simulink model "D_20210914_Modell_Inbetriebnahme_BreakOutBox_Jetson"  (R2021a)
(part 5 of 7)

  CAN Unpack60/8 -> Terminator530/1
  CAN Unpack60/11 -> Bus Creator60/4  "RCS"
  CAN Unpack60/14 -> Terminator533/1
  CAN Unpack60/15 -> Bus Creator60/6  "Speed_Radial"
  CAN Unpack60/9 -> Terminator531/1
  CAN Unpack60/6 -> Terminator528/1
  CAN Unpack60/16 -> Bus Creator60/7  "CAN ID"
  CAN Unpack60/17 -> Bus Creator60/8  "Timestamp"
  Bus Creator60/1 -> Bus Creator1/60  "Data_059"
  CAN Unpack60/1 -> Bus Creator60/1  "AZ_Winkel"
  CAN Unpack61/3 -> Terminator534/1
  CAN Unpack61/2 -> Bus Creator61/2  "EL_Angle"
  CAN Unpack61/13 -> Terminator541/1
  CAN Unpack61/7 -> Terminator538/1
  CAN Unpack61/12 -> Bus Creator61/5  "Range"
  CAN Unpack61/10 -> Bus Creator61/3  "Mode_Signal"
  CAN Unpack61/4 -> Terminator535/1
  CAN Unpack61/5 -> Terminator536/1
  CAN Unpack61/8 -> Terminator539/1
  CAN Unpack61/11 -> Bus Creator61/4  "RCS"
  CAN Unpack61/14 -> Terminator542/1
  CAN Unpack61/15 -> Bus Creator61/6  "Speed_Radial"
  CAN Unpack61/9 -> Terminator540/1
  CAN Unpack61/6 -> Terminator537/1
  CAN Unpack61/16 -> Bus Creator61/7  "CAN ID"
  CAN Unpack61/17 -> Bus Creator61/8  "Timestamp"
  Bus Creator61/1 -> Bus Creator1/61  "Data_060"
  CAN Unpack61/1 -> Bus Creator61/1  "AZ_Winkel"
  CAN Unpack62/3 -> Terminator543/1
  CAN Unpack62/2 -> Bus Creator62/2  "EL_Angle"
  CAN Unpack62/13 -> Terminator550/1
  CAN Unpack62/7 -> Terminator547/1
  CAN Unpack62/12 -> Bus Creator62/5  "Range"
  CAN Unpack62/10 -> Bus Creator62/3  "Mode_Signal"
  CAN Unpack62/4 -> Terminator544/1
  CAN Unpack62/5 -> Terminator545/1
  CAN Unpack62/8 -> Terminator548/1
  CAN Unpack62/11 -> Bus Creator62/4  "RCS"
  CAN Unpack62/14 -> Terminator551/1
  CAN Unpack62/15 -> Bus Creator62/6  "Speed_Radial"
  CAN Unpack62/9 -> Terminator549/1
  CAN Unpack62/6 -> Terminator546/1
  CAN Unpack62/16 -> Bus Creator62/7  "CAN ID"
  CAN Unpack62/17 -> Bus Creator62/8  "Timestamp"
  Bus Creator62/1 -> Bus Creator1/62  "Data_061"
  CAN Unpack62/1 -> Bus Creator62/1  "AZ_Winkel"
  CAN Unpack63/3 -> Terminator552/1
  CAN Unpack63/2 -> Bus Creator63/2  "EL_Angle"
  CAN Unpack63/13 -> Terminator559/1
  CAN Unpack63/7 -> Terminator556/1
  CAN Unpack63/12 -> Bus Creator63/5  "Range"
  CAN Unpack63/10 -> Bus Creator63/3  "Mode_Signal"
  CAN Unpack63/4 -> Terminator553/1
  CAN Unpack63/5 -> Terminator554/1
  CAN Unpack63/8 -> Terminator557/1
  CAN Unpack63/11 -> Bus Creator63/4  "RCS"
  CAN Unpack63/14 -> Terminator560/1
  CAN Unpack63/15 -> Bus Creator63/6  "Speed_Radial"
  CAN Unpack63/9 -> Terminator558/1
  CAN Unpack63/6 -> Terminator555/1
  CAN Unpack63/16 -> Bus Creator63/7  "CAN ID"
  CAN Unpack63/17 -> Bus Creator63/8  "Timestamp"
  Bus Creator63/1 -> Bus Creator1/63  "Data_062"
  CAN Unpack63/1 -> Bus Creator63/1  "AZ_Winkel"
  CAN Unpack64/3 -> Terminator561/1
  CAN Unpack64/2 -> Bus Creator64/2  "EL_Angle"
  CAN Unpack64/13 -> Terminator568/1
  CAN Unpack64/7 -> Terminator565/1
  CAN Unpack64/12 -> Bus Creator64/5  "Range"
  CAN Unpack64/10 -> Bus Creator64/3  "Mode_Signal"
  CAN Unpack64/4 -> Terminator562/1
  CAN Unpack64/5 -> Terminator563/1
  CAN Unpack64/8 -> Terminator566/1
  CAN Unpack64/11 -> Bus Creator64/4  "RCS"
  CAN Unpack64/14 -> Terminator569/1
  CAN Unpack64/15 -> Bus Creator64/6  "Speed_Radial"
  CAN Unpack64/9 -> Terminator567/1
  CAN Unpack64/6 -> Terminator564/1
  CAN Unpack64/16 -> Bus Creator64/7  "CAN ID"
  CAN Unpack64/17 -> Bus Creator64/8  "Timestamp"
  Bus Creator64/1 -> Bus Creator1/64  "Data_063"
  CAN Unpack64/1 -> Bus Creator64/1  "AZ_Winkel"
  CAN Unpack65/3 -> Terminator570/1
  CAN Unpack65/2 -> Bus Creator65/2  "EL_Angle"
  CAN Unpack65/13 -> Terminator577/1
  CAN Unpack65/7 -> Terminator574/1
  CAN Unpack65/12 -> Bus Creator65/5  "Range"
  CAN Unpack65/10 -> Bus Creator65/3  "Mode_Signal"
  CAN Unpack65/4 -> Terminator571/1
  CAN Unpack65/5 -> Terminator572/1
  CAN Unpack65/8 -> Terminator575/1
  CAN Unpack65/11 -> Bus Creator65/4  "RCS"
  CAN Unpack65/14 -> Terminator578/1
  CAN Unpack65/15 -> Bus Creator65/6  "Speed_Radial"
  CAN Unpack65/9 -> Terminator576/1
  CAN Unpack65/6 -> Terminator573/1
  CAN Unpack65/16 -> Bus Creator65/7  "CAN ID"
  CAN Unpack65/17 -> Bus Creator65/8  "Timestamp"
  Bus Creator65/1 -> Bus Creator1/65  "Data_064"
  CAN Unpack65/1 -> Bus Creator65/1  "AZ_Winkel"
  CAN Unpack66/3 -> Terminator579/1
  CAN Unpack66/2 -> Bus Creator66/2  "EL_Angle"
  CAN Unpack66/13 -> Terminator586/1
  CAN Unpack66/7 -> Terminator583/1
  CAN Unpack66/12 -> Bus Creator66/5  "Range"
  CAN Unpack66/10 -> Bus Creator66/3  "Mode_Signal"
  CAN Unpack66/4 -> Terminator580/1
  CAN Unpack66/5 -> Terminator581/1
  CAN Unpack66/8 -> Terminator584/1
  CAN Unpack66/11 -> Bus Creator66/4  "RCS"
  CAN Unpack66/14 -> Terminator587/1
  CAN Unpack66/15 -> Bus Creator66/6  "Speed_Radial"
  CAN Unpack66/9 -> Terminator585/1
  CAN Unpack66/6 -> Terminator582/1
  CAN Unpack66/16 -> Bus Creator66/7  "CAN ID"
  CAN Unpack66/17 -> Bus Creator66/8  "Timestamp"
  Bus Creator66/1 -> Bus Creator1/66  "Data_065"
  CAN Unpack66/1 -> Bus Creator66/1  "AZ_Winkel"
  CAN Unpack67/3 -> Terminator588/1
  CAN Unpack67/2 -> Bus Creator67/2  "EL_Angle"
  CAN Unpack67/13 -> Terminator595/1
  CAN Unpack67/7 -> Terminator592/1
  CAN Unpack67/12 -> Bus Creator67/5  "Range"
  CAN Unpack67/10 -> Bus Creator67/3  "Mode_Signal"
  CAN Unpack67/4 -> Terminator589/1
  CAN Unpack67/5 -> Terminator590/1
  CAN Unpack67/8 -> Terminator593/1
  CAN Unpack67/11 -> Bus Creator67/4  "RCS"
  CAN Unpack67/14 -> Terminator596/1
  CAN Unpack67/15 -> Bus Creator67/6  "Speed_Radial"
  CAN Unpack67/9 -> Terminator594/1
  CAN Unpack67/6 -> Terminator591/1
  CAN Unpack67/16 -> Bus Creator67/7  "CAN ID"
  CAN Unpack67/17 -> Bus Creator67/8  "Timestamp"
  Bus Creator67/1 -> Bus Creator1/67  "Data_066"
  CAN Unpack67/1 -> Bus Creator67/1  "AZ_Winkel"
  CAN Unpack68/3 -> Terminator597/1
  CAN Unpack68/2 -> Bus Creator68/2  "EL_Angle"
  CAN Unpack68/13 -> Terminator604/1
  CAN Unpack68/7 -> Terminator601/1
  CAN Unpack68/12 -> Bus Creator68/5  "Range"
  CAN Unpack68/10 -> Bus Creator68/3  "Mode_Signal"
  CAN Unpack68/4 -> Terminator598/1
  CAN Unpack68/5 -> Terminator599/1
  CAN Unpack68/8 -> Terminator602/1
  CAN Unpack68/11 -> Bus Creator68/4  "RCS"
  CAN Unpack68/14 -> Terminator605/1
  CAN Unpack68/15 -> Bus Creator68/6  "Speed_Radial"
  CAN Unpack68/9 -> Terminator603/1
  CAN Unpack68/6 -> Terminator600/1
  CAN Unpack68/16 -> Bus Creator68/7  "CAN ID"
  CAN Unpack68/17 -> Bus Creator68/8  "Timestamp"
  Bus Creator68/1 -> Bus Creator1/68  "Data_067"
  CAN Unpack68/1 -> Bus Creator68/1  "AZ_Winkel"
  CAN Unpack69/3 -> Terminator606/1
  CAN Unpack69/2 -> Bus Creator69/2  "EL_Angle"
  CAN Unpack69/13 -> Terminator613/1
  CAN Unpack69/7 -> Terminator610/1
  CAN Unpack69/12 -> Bus Creator69/5  "Range"
  CAN Unpack69/10 -> Bus Creator69/3  "Mode_Signal"
  CAN Unpack69/4 -> Terminator607/1
  CAN Unpack69/5 -> Terminator608/1
  CAN Unpack69/8 -> Terminator611/1
  CAN Unpack69/11 -> Bus Creator69/4  "RCS"
  CAN Unpack69/14 -> Terminator614/1
  CAN Unpack69/15 -> Bus Creator69/6  "Speed_Radial"
  CAN Unpack69/9 -> Terminator612/1
  CAN Unpack69/6 -> Terminator609/1
  CAN Unpack69/16 -> Bus Creator69/7  "CAN ID"
  CAN Unpack69/17 -> Bus Creator69/8  "Timestamp"
  Bus Creator69/1 -> Bus Creator1/69  "Data_068"
  CAN Unpack69/1 -> Bus Creator69/1  "AZ_Winkel"
  CAN Unpack70/3 -> Terminator615/1
  CAN Unpack70/2 -> Bus Creator70/2  "EL_Angle"
  CAN Unpack70/13 -> Terminator622/1
  CAN Unpack70/7 -> Terminator619/1
  CAN Unpack70/12 -> Bus Creator70/5  "Range"
  CAN Unpack70/10 -> Bus Creator70/3  "Mode_Signal"
  CAN Unpack70/4 -> Terminator616/1
  CAN Unpack70/5 -> Terminator617/1
  CAN Unpack70/8 -> Terminator620/1
  CAN Unpack70/11 -> Bus Creator70/4  "RCS"
  CAN Unpack70/14 -> Terminator623/1
  CAN Unpack70/15 -> Bus Creator70/6  "Speed_Radial"
  CAN Unpack70/9 -> Terminator621/1
  CAN Unpack70/6 -> Terminator618/1
  CAN Unpack70/16 -> Bus Creator70/7  "CAN ID"
  CAN Unpack70/17 -> Bus Creator70/8  "Timestamp"
  Bus Creator70/1 -> Bus Creator1/70  "Data_069"
  CAN Unpack70/1 -> Bus Creator70/1  "AZ_Winkel"
  CAN Unpack71/3 -> Terminator624/1
  CAN Unpack71/2 -> Bus Creator71/2  "EL_Angle"
  CAN Unpack71/13 -> Terminator631/1
  CAN Unpack71/7 -> Terminator628/1
  CAN Unpack71/12 -> Bus Creator71/5  "Range"
  CAN Unpack71/10 -> Bus Creator71/3  "Mode_Signal"
  CAN Unpack71/4 -> Terminator625/1
  CAN Unpack71/5 -> Terminator626/1
  CAN Unpack71/8 -> Terminator629/1
  CAN Unpack71/11 -> Bus Creator71/4  "RCS"
  CAN Unpack71/14 -> Terminator632/1
  CAN Unpack71/15 -> Bus Creator71/6  "Speed_Radial"
  CAN Unpack71/9 -> Terminator630/1
  CAN Unpack71/6 -> Terminator627/1
  CAN Unpack71/16 -> Bus Creator71/7  "CAN ID"
  CAN Unpack71/17 -> Bus Creator71/8  "Timestamp"
  Bus Creator71/1 -> Bus Creator1/71  "Data_070"
  CAN Unpack71/1 -> Bus Creator71/1  "AZ_Winkel"
  CAN Unpack72/3 -> Terminator633/1
  CAN Unpack72/2 -> Bus Creator72/2  "EL_Angle"
  CAN Unpack72/13 -> Terminator640/1
  CAN Unpack72/7 -> Terminator637/1
  CAN Unpack72/12 -> Bus Creator72/5  "Range"
  CAN Unpack72/10 -> Bus Creator72/3  "Mode_Signal"
  CAN Unpack72/4 -> Terminator634/1
  CAN Unpack72/5 -> Terminator635/1
  CAN Unpack72/8 -> Terminator638/1
  CAN Unpack72/11 -> Bus Creator72/4  "RCS"
  CAN Unpack72/14 -> Terminator641/1
  CAN Unpack72/15 -> Bus Creator72/6  "Speed_Radial"
  CAN Unpack72/9 -> Terminator639/1
  CAN Unpack72/6 -> Terminator636/1
  CAN Unpack72/16 -> Bus Creator72/7  "CAN ID"
  CAN Unpack72/17 -> Bus Creator72/8  "Timestamp"
  Bus Creator72/1 -> Bus Creator1/72  "Data_071"
  CAN Unpack72/1 -> Bus Creator72/1  "AZ_Winkel"
  CAN Unpack73/3 -> Terminator642/1
  CAN Unpack73/2 -> Bus Creator73/2  "EL_Angle"
  CAN Unpack73/13 -> Terminator649/1
  CAN Unpack73/7 -> Terminator646/1
  CAN Unpack73/12 -> Bus Creator73/5  "Range"
  CAN Unpack73/10 -> Bus Creator73/3  "Mode_Signal"
  CAN Unpack73/4 -> Terminator643/1
  CAN Unpack73/5 -> Terminator644/1
  CAN Unpack73/8 -> Terminator647/1
  CAN Unpack73/11 -> Bus Creator73/4  "RCS"
  CAN Unpack73/14 -> Terminator650/1
  CAN Unpack73/15 -> Bus Creator73/6  "Speed_Radial"
  CAN Unpack73/9 -> Terminator648/1
  CAN Unpack73/6 -> Terminator645/1
  CAN Unpack73/16 -> Bus Creator73/7  "CAN ID"
  CAN Unpack73/17 -> Bus Creator73/8  "Timestamp"
  Bus Creator73/1 -> Bus Creator1/73  "Data_072"
  CAN Unpack73/1 -> Bus Creator73/1  "AZ_Winkel"
  CAN Unpack74/3 -> Terminator651/1
  CAN Unpack74/2 -> Bus Creator74/2  "EL_Angle"
  CAN Unpack74/13 -> Terminator658/1
  CAN Unpack74/7 -> Terminator655/1
  CAN Unpack74/12 -> Bus Creator74/5  "Range"
  CAN Unpack74/10 -> Bus Creator74/3  "Mode_Signal"
  CAN Unpack74/4 -> Terminator652/1
  CAN Unpack74/5 -> Terminator653/1
  CAN Unpack74/8 -> Terminator656/1
  CAN Unpack74/11 -> Bus Creator74/4  "RCS"
  CAN Unpack74/14 -> Terminator659/1
  CAN Unpack74/15 -> Bus Creator74/6  "Speed_Radial"
  CAN Unpack74/9 -> Terminator657/1
  CAN Unpack74/6 -> Terminator654/1
  CAN Unpack74/16 -> Bus Creator74/7  "CAN ID"
  CAN Unpack74/17 -> Bus Creator74/8  "Timestamp"
  Bus Creator74/1 -> Bus Creator1/74  "Data_073"
  CAN Unpack74/1 -> Bus Creator74/1  "AZ_Winkel"
  CAN Unpack75/3 -> Terminator660/1
  CAN Unpack75/2 -> Bus Creator75/2  "EL_Angle"
  CAN Unpack75/13 -> Terminator667/1
  CAN Unpack75/7 -> Terminator664/1
  CAN Unpack75/12 -> Bus Creator75/5  "Range"
  CAN Unpack75/10 -> Bus Creator75/3  "Mode_Signal"
  CAN Unpack75/4 -> Terminator661/1
  CAN Unpack75/5 -> Terminator662/1
  CAN Unpack75/8 -> Terminator665/1
  CAN Unpack75/11 -> Bus Creator75/4  "RCS"
  CAN Unpack75/14 -> Terminator668/1
  CAN Unpack75/15 -> Bus Creator75/6  "Speed_Radial"
  CAN Unpack75/9 -> Terminator666/1
  CAN Unpack75/6 -> Terminator663/1
  CAN Unpack75/16 -> Bus Creator75/7  "CAN ID"
  CAN Unpack75/17 -> Bus Creator75/8  "Timestamp"
  Bus Creator75/1 -> Bus Creator1/75  "Data_074"
  CAN Unpack75/1 -> Bus Creator75/1  "AZ_Winkel"
  CAN Unpack76/3 -> Terminator669/1
  CAN Unpack76/2 -> Bus Creator76/2  "EL_Angle"
  CAN Unpack76/13 -> Terminator676/1
  CAN Unpack76/7 -> Terminator673/1
  CAN Unpack76/12 -> Bus Creator76/5  "Range"
  CAN Unpack76/10 -> Bus Creator76/3  "Mode_Signal"
  CAN Unpack76/4 -> Terminator670/1
  CAN Unpack76/5 -> Terminator671/1
  CAN Unpack76/8 -> Terminator674/1
  CAN Unpack76/11 -> Bus Creator76/4  "RCS"
  CAN Unpack76/14 -> Terminator677/1
  CAN Unpack76/15 -> Bus Creator76/6  "Speed_Radial"
  CAN Unpack76/9 -> Terminator675/1
  CAN Unpack76/6 -> Terminator672/1
  CAN Unpack76/16 -> Bus Creator76/7  "CAN ID"
  CAN Unpack76/17 -> Bus Creator76/8  "Timestamp"
  Bus Creator76/1 -> Bus Creator1/76  "Data_075"
  CAN Unpack76/1 -> Bus Creator76/1  "AZ_Winkel"
  CAN Unpack77/3 -> Terminator678/1
  CAN Unpack77/2 -> Bus Creator77/2  "EL_Angle"
  CAN Unpack77/13 -> Terminator685/1
  CAN Unpack77/7 -> Terminator682/1
  CAN Unpack77/12 -> Bus Creator77/5  "Range"
  CAN Unpack77/10 -> Bus Creator77/3  "Mode_Signal"
  CAN Unpack77/4 -> Terminator679/1
  CAN Unpack77/5 -> Terminator680/1
  CAN Unpack77/8 -> Terminator683/1
  CAN Unpack77/11 -> Bus Creator77/4  "RCS"
  CAN Unpack77/14 -> Terminator686/1
  CAN Unpack77/15 -> Bus Creator77/6  "Speed_Radial"
  CAN Unpack77/9 -> Terminator684/1
  CAN Unpack77/6 -> Terminator681/1
  CAN Unpack77/16 -> Bus Creator77/7  "CAN ID"
  CAN Unpack77/17 -> Bus Creator77/8  "Timestamp"
  Bus Creator77/1 -> Bus Creator1/77  "Data_076"
  CAN Unpack77/1 -> Bus Creator77/1  "AZ_Winkel"
  CAN Unpack78/3 -> Terminator687/1
  CAN Unpack78/2 -> Bus Creator78/2  "EL_Angle"
  CAN Unpack78/13 -> Terminator694/1
  CAN Unpack78/7 -> Terminator691/1
  CAN Unpack78/12 -> Bus Creator78/5  "Range"
  CAN Unpack78/10 -> Bus Creator78/3  "Mode_Signal"
  CAN Unpack78/4 -> Terminator688/1
  CAN Unpack78/5 -> Terminator689/1
  CAN Unpack78/8 -> Terminator692/1
  CAN Unpack78/11 -> Bus Creator78/4  "RCS"
  CAN Unpack78/14 -> Terminator695/1
  CAN Unpack78/15 -> Bus Creator78/6  "Speed_Radial"
  CAN Unpack78/9 -> Terminator693/1
  CAN Unpack78/6 -> Terminator690/1
  CAN Unpack78/16 -> Bus Creator78/7  "CAN ID"
  CAN Unpack78/17 -> Bus Creator78/8  "Timestamp"
  Bus Creator78/1 -> Bus Creator1/78  "Data_077"
  CAN Unpack78/1 -> Bus Creator78/1  "AZ_Winkel"
  CAN Unpack79/3 -> Terminator696/1
  CAN Unpack79/2 -> Bus Creator79/2  "EL_Angle"
  CAN Unpack79/13 -> Terminator703/1
  CAN Unpack79/7 -> Terminator700/1
  CAN Unpack79/12 -> Bus Creator79/5  "Range"
  CAN Unpack79/10 -> Bus Creator79/3  "Mode_Signal"
  CAN Unpack79/4 -> Terminator697/1
  CAN Unpack79/5 -> Terminator698/1
  CAN Unpack79/8 -> Terminator701/1
  CAN Unpack79/11 -> Bus Creator79/4  "RCS"
  CAN Unpack79/14 -> Terminator704/1
  CAN Unpack79/15 -> Bus Creator79/6  "Speed_Radial"
  CAN Unpack79/9 -> Terminator702/1
  CAN Unpack79/6 -> Terminator699/1
  CAN Unpack79/16 -> Bus Creator79/7  "CAN ID"
  CAN Unpack79/17 -> Bus Creator79/8  "Timestamp"
  Bus Creator79/1 -> Bus Creator1/79  "Data_078"
  CAN Unpack79/1 -> Bus Creator79/1  "AZ_Winkel"
  CAN Unpack80/3 -> Terminator705/1
  CAN Unpack80/2 -> Bus Creator80/2  "EL_Angle"
  CAN Unpack80/13 -> Terminator712/1
  CAN Unpack80/7 -> Terminator709/1
  CAN Unpack80/12 -> Bus Creator80/5  "Range"
  CAN Unpack80/10 -> Bus Creator80/3  "Mode_Signal"
  CAN Unpack80/4 -> Terminator706/1
  CAN Unpack80/5 -> Terminator707/1
  CAN Unpack80/8 -> Terminator710/1
  CAN Unpack80/11 -> Bus Creator80/4  "RCS"
  CAN Unpack80/14 -> Terminator713/1
  CAN Unpack80/15 -> Bus Creator80/6  "Speed_Radial"
  CAN Unpack80/9 -> Terminator711/1
  CAN Unpack80/6 -> Terminator708/1
  CAN Unpack80/16 -> Bus Creator80/7  "CAN ID"
  CAN Unpack80/17 -> Bus Creator80/8  "Timestamp"
  Bus Creator80/1 -> Bus Creator1/80  "Data_079"
  CAN Unpack80/1 -> Bus Creator80/1  "AZ_Winkel"
  CAN Unpack81/3 -> Terminator714/1
  CAN Unpack81/2 -> Bus Creator81/2  "EL_Angle"
  CAN Unpack81/13 -> Terminator721/1
  CAN Unpack81/7 -> Terminator718/1
  CAN Unpack81/12 -> Bus Creator81/5  "Range"
  CAN Unpack81/10 -> Bus Creator81/3  "Mode_Signal"
  CAN Unpack81/4 -> Terminator715/1
  CAN Unpack81/5 -> Terminator716/1
  CAN Unpack81/8 -> Terminator719/1
  CAN Unpack81/11 -> Bus Creator81/4  "RCS"
  CAN Unpack81/14 -> Terminator722/1
  CAN Unpack81/15 -> Bus Creator81/6  "Speed_Radial"
  CAN Unpack81/9 -> Terminator720/1
  CAN Unpack81/6 -> Terminator717/1
  CAN Unpack81/16 -> Bus Creator81/7  "CAN ID"
  CAN Unpack81/17 -> Bus Creator81/8  "Timestamp"
  Bus Creator81/1 -> Bus Creator1/81  "Data_080"
  CAN Unpack81/1 -> Bus Creator81/1  "AZ_Winkel"
  CAN Unpack82/3 -> Terminator723/1
  CAN Unpack82/2 -> Bus Creator82/2  "EL_Angle"
  CAN Unpack82/13 -> Terminator730/1
  CAN Unpack82/7 -> Terminator727/1
  CAN Unpack82/12 -> Bus Creator82/5  "Range"
  CAN Unpack82/10 -> Bus Creator82/3  "Mode_Signal"
  CAN Unpack82/4 -> Terminator724/1
  CAN Unpack82/5 -> Terminator725/1
  CAN Unpack82/8 -> Terminator728/1
  CAN Unpack82/11 -> Bus Creator82/4  "RCS"
  CAN Unpack82/14 -> Terminator731/1
  CAN Unpack82/15 -> Bus Creator82/6  "Speed_Radial"
  CAN Unpack82/9 -> Terminator729/1
  CAN Unpack82/6 -> Terminator726/1
  CAN Unpack82/16 -> Bus Creator82/7  "CAN ID"
  CAN Unpack82/17 -> Bus Creator82/8  "Timestamp"
  Bus Creator82/1 -> Bus Creator1/82  "Data_081"
  CAN Unpack82/1 -> Bus Creator82/1  "AZ_Winkel"
  CAN Unpack83/3 -> Terminator732/1
  CAN Unpack83/2 -> Bus Creator83/2  "EL_Angle"
  CAN Unpack83/13 -> Terminator739/1
  CAN Unpack83/7 -> Terminator736/1
  CAN Unpack83/12 -> Bus Creator83/5  "Range"
  CAN Unpack83/10 -> Bus Creator83/3  "Mode_Signal"
  CAN Unpack83/4 -> Terminator733/1
  CAN Unpack83/5 -> Terminator734/1
  CAN Unpack83/8 -> Terminator737/1
  CAN Unpack83/11 -> Bus Creator83/4  "RCS"
  CAN Unpack83/14 -> Terminator740/1
  CAN Unpack83/15 -> Bus Creator83/6  "Speed_Radial"
  CAN Unpack83/9 -> Terminator738/1
  CAN Unpack83/6 -> Terminator735/1
  CAN Unpack83/16 -> Bus Creator83/7  "CAN ID"
  CAN Unpack83/17 -> Bus Creator83/8  "Timestamp"
  Bus Creator83/1 -> Bus Creator1/83  "Data_082"
  CAN Unpack83/1 -> Bus Creator83/1  "AZ_Winkel"
  CAN Unpack84/3 -> Terminator741/1
  CAN Unpack84/2 -> Bus Creator84/2  "EL_Angle"
  CAN Unpack84/13 -> Terminator748/1
  CAN Unpack84/7 -> Terminator745/1
  CAN Unpack84/12 -> Bus Creator84/5  "Range"
  CAN Unpack84/10 -> Bus Creator84/3  "Mode_Signal"
  CAN Unpack84/4 -> Terminator742/1
  CAN Unpack84/5 -> Terminator743/1
  CAN Unpack84/8 -> Terminator746/1
  CAN Unpack84/11 -> Bus Creator84/4  "RCS"
  CAN Unpack84/14 -> Terminator749/1
  CAN Unpack84/15 -> Bus Creator84/6  "Speed_Radial"
  CAN Unpack84/9 -> Terminator747/1
  CAN Unpack84/6 -> Terminator744/1
  CAN Unpack84/16 -> Bus Creator84/7  "CAN ID"
  CAN Unpack84/17 -> Bus Creator84/8  "Timestamp"
  Bus Creator84/1 -> Bus Creator1/84  "Data_083"
  CAN Unpack84/1 -> Bus Creator84/1  "AZ_Winkel"
  CAN Unpack85/3 -> Terminator750/1
  CAN Unpack85/2 -> Bus Creator85/2  "EL_Angle"
  CAN Unpack85/13 -> Terminator757/1
  CAN Unpack85/7 -> Terminator754/1
  CAN Unpack85/12 -> Bus Creator85/5  "Range"
  CAN Unpack85/10 -> Bus Creator85/3  "Mode_Signal"
  CAN Unpack85/4 -> Terminator751/1
  CAN Unpack85/5 -> Terminator752/1
  CAN Unpack85/8 -> Terminator755/1
  CAN Unpack85/11 -> Bus Creator85/4  "RCS"
  CAN Unpack85/14 -> Terminator758/1
  CAN Unpack85/15 -> Bus Creator85/6  "Speed_Radial"
  CAN Unpack85/9 -> Terminator756/1
  CAN Unpack85/6 -> Terminator753/1
  CAN Unpack85/16 -> Bus Creator85/7  "CAN ID"
  CAN Unpack85/17 -> Bus Creator85/8  "Timestamp"
  Bus Creator85/1 -> Bus Creator1/85  "Data_084"
  CAN Unpack85/1 -> Bus Creator85/1  "AZ_Winkel"
  CAN Unpack86/3 -> Terminator759/1
  CAN Unpack86/2 -> Bus Creator86/2  "EL_Angle"
  CAN Unpack86/13 -> Terminator766/1
  CAN Unpack86/7 -> Terminator763/1
  CAN Unpack86/12 -> Bus Creator86/5  "Range"
  CAN Unpack86/10 -> Bus Creator86/3  "Mode_Signal"
  CAN Unpack86/4 -> Terminator760/1
  CAN Unpack86/5 -> Terminator761/1
  CAN Unpack86/8 -> Terminator764/1
  CAN Unpack86/11 -> Bus Creator86/4  "RCS"
  CAN Unpack86/14 -> Terminator767/1
  CAN Unpack86/15 -> Bus Creator86/6  "Speed_Radial"
  CAN Unpack86/9 -> Terminator765/1
  CAN Unpack86/6 -> Terminator762/1
  CAN Unpack86/16 -> Bus Creator86/7  "CAN ID"
  CAN Unpack86/17 -> Bus Creator86/8  "Timestamp"
  Bus Creator86/1 -> Bus Creator1/86  "Data_085"
  CAN Unpack86/1 -> Bus Creator86/1  "AZ_Winkel"
  CAN Unpack87/3 -> Terminator768/1
  CAN Unpack87/2 -> Bus Creator87/2  "EL_Angle"
  CAN Unpack87/13 -> Terminator775/1
  CAN Unpack87/7 -> Terminator772/1
  CAN Unpack87/12 -> Bus Creator87/5  "Range"
  CAN Unpack87/10 -> Bus Creator87/3  "Mode_Signal"
  CAN Unpack87/4 -> Terminator769/1
  CAN Unpack87/5 -> Terminator770/1
  CAN Unpack87/8 -> Terminator773/1
  CAN Unpack87/11 -> Bus Creator87/4  "RCS"
  CAN Unpack87/14 -> Terminator776/1
  CAN Unpack87/15 -> Bus Creator87/6  "Speed_Radial"
  CAN Unpack87/9 -> Terminator774/1
  CAN Unpack87/6 -> Terminator771/1
  CAN Unpack87/16 -> Bus Creator87/7  "CAN ID"
  CAN Unpack87/17 -> Bus Creator87/8  "Timestamp"
  Bus Creator87/1 -> Bus Creator1/87  "Data_086"
  CAN Unpack87/1 -> Bus Creator87/1  "AZ_Winkel"
  CAN Unpack88/3 -> Terminator777/1
  CAN Unpack88/2 -> Bus Creator88/2  "EL_Angle"
  CAN Unpack88/13 -> Terminator784/1
  CAN Unpack88/7 -> Terminator781/1
  CAN Unpack88/12 -> Bus Creator88/5  "Range"
  CAN Unpack88/10 -> Bus Creator88/3  "Mode_Signal"
  CAN Unpack88/4 -> Terminator778/1
  CAN Unpack88/5 -> Terminator779/1
  CAN Unpack88/8 -> Terminator782/1
  CAN Unpack88/11 -> Bus Creator88/4  "RCS"
  CAN Unpack88/14 -> Terminator785/1
  CAN Unpack88/15 -> Bus Creator88/6  "Speed_Radial"
  CAN Unpack88/9 -> Terminator783/1
  CAN Unpack88/6 -> Terminator780/1
  CAN Unpack88/16 -> Bus Creator88/7  "CAN ID"
  CAN Unpack88/17 -> Bus Creator88/8  "Timestamp"
  Bus Creator88/1 -> Bus Creator1/88  "Data_087"
  CAN Unpack88/1 -> Bus Creator88/1  "AZ_Winkel"
  CAN Unpack89/3 -> Terminator786/1
  CAN Unpack89/2 -> Bus Creator89/2  "EL_Angle"
  CAN Unpack89/13 -> Terminator793/1
  CAN Unpack89/7 -> Terminator790/1
  CAN Unpack89/12 -> Bus Creator89/5  "Range"
  CAN Unpack89/10 -> Bus Creator89/3  "Mode_Signal"
  CAN Unpack89/4 -> Terminator787/1
  CAN Unpack89/5 -> Terminator788/1
  CAN Unpack89/8 -> Terminator791/1
  CAN Unpack89/11 -> Bus Creator89/4  "RCS"
  CAN Unpack89/14 -> Terminator794/1
  CAN Unpack89/15 -> Bus Creator89/6  "Speed_Radial"
  CAN Unpack89/9 -> Terminator792/1
  CAN Unpack89/6 -> Terminator789/1
  CAN Unpack89/16 -> Bus Creator89/7  "CAN ID"
  CAN Unpack89/17 -> Bus Creator89/8  "Timestamp"
  Bus Creator89/1 -> Bus Creator1/89  "Data_088"
  CAN Unpack89/1 -> Bus Creator89/1  "AZ_Winkel"
  CAN Unpack90/3 -> Terminator795/1
  CAN Unpack90/2 -> Bus Creator90/2  "EL_Angle"
  CAN Unpack90/13 -> Terminator802/1
  CAN Unpack90/7 -> Terminator799/1
  CAN Unpack90/12 -> Bus Creator90/5  "Range"
  CAN Unpack90/10 -> Bus Creator90/3  "Mode_Signal"
  CAN Unpack90/4 -> Terminator796/1
  CAN Unpack90/5 -> Terminator797/1
  CAN Unpack90/8 -> Terminator800/1
  CAN Unpack90/11 -> Bus Creator90/4  "RCS"
  CAN Unpack90/14 -> Terminator803/1
  CAN Unpack90/15 -> Bus Creator90/6  "Speed_Radial"
  CAN Unpack90/9 -> Terminator801/1
  CAN Unpack90/6 -> Terminator798/1
  CAN Unpack90/16 -> Bus Creator90/7  "CAN ID"
  CAN Unpack90/17 -> Bus Creator90/8  "Timestamp"
  Bus Creator90/1 -> Bus Creator1/90  "Data_089"
  CAN Unpack90/1 -> Bus Creator90/1  "AZ_Winkel"
  CAN Unpack91/3 -> Terminator804/1
  CAN Unpack91/2 -> Bus Creator91/2  "EL_Angle"
  CAN Unpack91/13 -> Terminator811/1
  CAN Unpack91/7 -> Terminator808/1
  CAN Unpack91/12 -> Bus Creator91/5  "Range"
  CAN Unpack91/10 -> Bus Creator91/3  "Mode_Signal"
  CAN Unpack91/4 -> Terminator805/1
  CAN Unpack91/5 -> Terminator806/1
  CAN Unpack91/8 -> Terminator809/1
  CAN Unpack91/11 -> Bus Creator91/4  "RCS"
  CAN Unpack91/14 -> Terminator812/1
  CAN Unpack91/15 -> Bus Creator91/6  "Speed_Radial"
  CAN Unpack91/9 -> Terminator810/1
  CAN Unpack91/6 -> Terminator807/1
  CAN Unpack91/16 -> Bus Creator91/7  "CAN ID"
  CAN Unpack91/17 -> Bus Creator91/8  "Timestamp"
  Bus Creator91/1 -> Bus Creator1/91  "Data_090"
  CAN Unpack91/1 -> Bus Creator91/1  "AZ_Winkel"
  CAN Unpack92/3 -> Terminator813/1
  CAN Unpack92/2 -> Bus Creator92/2  "EL_Angle"
  CAN Unpack92/13 -> Terminator820/1
  CAN Unpack92/7 -> Terminator817/1
  CAN Unpack92/12 -> Bus Creator92/5  "Range"
  CAN Unpack92/10 -> Bus Creator92/3  "Mode_Signal"
  CAN Unpack92/4 -> Terminator814/1
  CAN Unpack92/5 -> Terminator815/1
  CAN Unpack92/8 -> Terminator818/1
  CAN Unpack92/11 -> Bus Creator92/4  "RCS"
  CAN Unpack92/14 -> Terminator821/1
  CAN Unpack92/15 -> Bus Creator92/6  "Speed_Radial"
  CAN Unpack92/9 -> Terminator819/1
  CAN Unpack92/6 -> Terminator816/1
  CAN Unpack92/16 -> Bus Creator92/7  "CAN ID"
  CAN Unpack92/17 -> Bus Creator92/8  "Timestamp"
  Bus Creator92/1 -> Bus Creator1/92  "Data_091"
  CAN Unpack92/1 -> Bus Creator92/1  "AZ_Winkel"
  CAN Unpack93/3 -> Terminator822/1
  CAN Unpack93/2 -> Bus Creator93/2  "EL_Angle"
  CAN Unpack93/13 -> Terminator829/1
  CAN Unpack93/7 -> Terminator826/1
  CAN Unpack93/12 -> Bus Creator93/5  "Range"
  CAN Unpack93/10 -> Bus Creator93/3  "Mode_Signal"
  CAN Unpack93/4 -> Terminator823/1
  CAN Unpack93/5 -> Terminator824/1
  CAN Unpack93/8 -> Terminator827/1
  CAN Unpack93/11 -> Bus Creator93/4  "RCS"
  CAN Unpack93/14 -> Terminator830/1
  CAN Unpack93/15 -> Bus Creator93/6  "Speed_Radial"
  CAN Unpack93/9 -> Terminator828/1
  CAN Unpack93/6 -> Terminator825/1
  CAN Unpack93/16 -> Bus Creator93/7  "CAN ID"
  CAN Unpack93/17 -> Bus Creator93/8  "Timestamp"
  Bus Creator93/1 -> Bus Creator1/93  "Data_092"
  CAN Unpack93/1 -> Bus Creator93/1  "AZ_Winkel"
  CAN Unpack94/3 -> Terminator831/1
  CAN Unpack94/2 -> Bus Creator94/2  "EL_Angle"
  CAN Unpack94/13 -> Terminator838/1
  CAN Unpack94/7 -> Terminator835/1
  CAN Unpack94/12 -> Bus Creator94/5  "Range"
  CAN Unpack94/10 -> Bus Creator94/3  "Mode_Signal"
  CAN Unpack94/4 -> Terminator832/1
  CAN Unpack94/5 -> Terminator833/1
  CAN Unpack94/8 -> Terminator836/1
  CAN Unpack94/11 -> Bus Creator94/4  "RCS"
  CAN Unpack94/14 -> Terminator839/1
  CAN Unpack94/15 -> Bus Creator94/6  "Speed_Radial"
  CAN Unpack94/9 -> Terminator837/1
  CAN Unpack94/6 -> Terminator834/1
  CAN Unpack94/16 -> Bus Creator94/7  "CAN ID"
  CAN Unpack94/17 -> Bus Creator94/8  "Timestamp"
  Bus Creator94/1 -> Bus Creator1/94  "Data_093"
  CAN Unpack94/1 -> Bus Creator94/1  "AZ_Winkel"
  CAN Unpack95/3 -> Terminator840/1
  CAN Unpack95/2 -> Bus Creator95/2  "EL_Angle"
  CAN Unpack95/13 -> Terminator847/1
  CAN Unpack95/7 -> Terminator844/1
  CAN Unpack95/12 -> Bus Creator95/5  "Range"
  CAN Unpack95/10 -> Bus Creator95/3  "Mode_Signal"
  CAN Unpack95/4 -> Terminator841/1
  CAN Unpack95/5 -> Terminator842/1
  CAN Unpack95/8 -> Terminator845/1
  CAN Unpack95/11 -> Bus Creator95/4  "RCS"
  CAN Unpack95/14 -> Terminator848/1
  CAN Unpack95/15 -> Bus Creator95/6  "Speed_Radial"
  CAN Unpack95/9 -> Terminator846/1
  CAN Unpack95/6 -> Terminator843/1
  CAN Unpack95/16 -> Bus Creator95/7  "CAN ID"
  CAN Unpack95/17 -> Bus Creator95/8  "Timestamp"
  Bus Creator95/1 -> Bus Creator1/95  "Data_094"
  CAN Unpack95/1 -> Bus Creator95/1  "AZ_Winkel"
  CAN Unpack96/3 -> Terminator849/1
  CAN Unpack96/2 -> Bus Creator96/2  "EL_Angle"
  CAN Unpack96/13 -> Terminator856/1
  CAN Unpack96/7 -> Terminator853/1
  CAN Unpack96/12 -> Bus Creator96/5  "Range"
  CAN Unpack96/10 -> Bus Creator96/3  "Mode_Signal"
  CAN Unpack96/4 -> Terminator850/1
  CAN Unpack96/5 -> Terminator851/1
  CAN Unpack96/8 -> Terminator854/1
  CAN Unpack96/11 -> Bus Creator96/4  "RCS"
  CAN Unpack96/14 -> Terminator857/1
  CAN Unpack96/15 -> Bus Creator96/6  "Speed_Radial"
  CAN Unpack96/9 -> Terminator855/1
  CAN Unpack96/6 -> Terminator852/1
  CAN Unpack96/16 -> Bus Creator96/7  "CAN ID"
  CAN Unpack96/17 -> Bus Creator96/8  "Timestamp"
  Bus Creator96/1 -> Bus Creator1/96  "Data_095"
  CAN Unpack96/1 -> Bus Creator96/1  "AZ_Winkel"
  CAN Unpack97/3 -> Terminator858/1
  CAN Unpack97/2 -> Bus Creator97/2  "EL_Angle"
  CAN Unpack97/13 -> Terminator865/1
  CAN Unpack97/7 -> Terminator862/1
  CAN Unpack97/12 -> Bus Creator97/5  "Range"
  CAN Unpack97/10 -> Bus Creator97/3  "Mode_Signal"
  CAN Unpack97/4 -> Terminator859/1
  CAN Unpack97/5 -> Terminator860/1
  CAN Unpack97/8 -> Terminator863/1
  CAN Unpack97/11 -> Bus Creator97/4  "RCS"
  CAN Unpack97/14 -> Terminator866/1
  CAN Unpack97/15 -> Bus Creator97/6  "Speed_Radial"
  CAN Unpack97/9 -> Terminator864/1
  CAN Unpack97/6 -> Terminator861/1
  CAN Unpack97/16 -> Bus Creator97/7  "CAN ID"
  CAN Unpack97/17 -> Bus Creator97/8  "Timestamp"
  Bus Creator97/1 -> Bus Creator1/97  "Data_096"
  CAN Unpack97/1 -> Bus Creator97/1  "AZ_Winkel"
  CAN Unpack98/3 -> Terminator867/1
  CAN Unpack98/2 -> Bus Creator98/2  "EL_Angle"
  CAN Unpack98/13 -> Terminator874/1
  CAN Unpack98/7 -> Terminator871/1
  CAN Unpack98/12 -> Bus Creator98/5  "Range"
  CAN Unpack98/10 -> Bus Creator98/3  "Mode_Signal"
  CAN Unpack98/4 -> Terminator868/1
  CAN Unpack98/5 -> Terminator869/1
  CAN Unpack98/8 -> Terminator872/1
  CAN Unpack98/11 -> Bus Creator98/4  "RCS"
  CAN Unpack98/14 -> Terminator875/1
  CAN Unpack98/15 -> Bus Creator98/6  "Speed_Radial"
  CAN Unpack98/9 -> Terminator873/1
  CAN Unpack98/6 -> Terminator870/1
  CAN Unpack98/16 -> Bus Creator98/7  "CAN ID"
  CAN Unpack98/17 -> Bus Creator98/8  "Timestamp"
  Bus Creator98/1 -> Bus Creator1/98  "Data_097"
  CAN Unpack98/1 -> Bus Creator98/1  "AZ_Winkel"
  CAN Unpack99/3 -> Terminator876/1
  CAN Unpack99/2 -> Bus Creator99/2  "EL_Angle"
  CAN Unpack99/13 -> Terminator883/1
  CAN Unpack99/7 -> Terminator880/1
  CAN Unpack99/12 -> Bus Creator99/5  "Range"
  CAN Unpack99/10 -> Bus Creator99/3  "Mode_Signal"
  CAN Unpack99/4 -> Terminator877/1
  CAN Unpack99/5 -> Terminator878/1
  CAN Unpack99/8 -> Terminator881/1
  CAN Unpack99/11 -> Bus Creator99/4  "RCS"
  CAN Unpack99/14 -> Terminator884/1
  CAN Unpack99/15 -> Bus Creator99/6  "Speed_Radial"
  CAN Unpack99/9 -> Terminator882/1
  CAN Unpack99/6 -> Terminator879/1
  CAN Unpack99/16 -> Bus Creator99/7  "CAN ID"
  CAN Unpack99/17 -> Bus Creator99/8  "Timestamp"
  Bus Creator99/1 -> Bus Creator1/99  "Data_098"
  CAN Unpack99/1 -> Bus Creator99/1  "AZ_Winkel"
  CAN Unpack100/3 -> Terminator885/1
  CAN Unpack100/2 -> Bus Creator100/2  "EL_Angle"
  CAN Unpack100/13 -> Terminator892/1
  CAN Unpack100/7 -> Terminator889/1
  CAN Unpack100/12 -> Bus Creator100/5  "Range"
  CAN Unpack100/10 -> Bus Creator100/3  "Mode_Signal"
  CAN Unpack100/4 -> Terminator886/1
  CAN Unpack100/5 -> Terminator887/1
  CAN Unpack100/8 -> Terminator890/1
  CAN Unpack100/11 -> Bus Creator100/4  "RCS"
  CAN Unpack100/14 -> Terminator893/1
  CAN Unpack100/15 -> Bus Creator100/6  "Speed_Radial"
  CAN Unpack100/9 -> Terminator891/1
  CAN Unpack100/6 -> Terminator888/1
  CAN Unpack100/16 -> Bus Creator100/7  "CAN ID"
  CAN Unpack100/17 -> Bus Creator100/8  "Timestamp"
  Bus Creator100/1 -> Bus Creator1/100  "Data_099"
  CAN Unpack100/1 -> Bus Creator100/1  "AZ_Winkel"
  CAN Unpack101/3 -> Terminator894/1
  CAN Unpack101/2 -> Bus Creator101/2  "EL_Angle"
  CAN Unpack101/13 -> Terminator901/1
  CAN Unpack101/7 -> Terminator898/1
  CAN Unpack101/12 -> Bus Creator101/5  "Range"
  CAN Unpack101/10 -> Bus Creator101/3  "Mode_Signal"
  CAN Unpack101/4 -> Terminator895/1
  CAN Unpack101/5 -> Terminator896/1
  CAN Unpack101/8 -> Terminator899/1
  CAN Unpack101/11 -> Bus Creator101/4  "RCS"
  CAN Unpack101/14 -> Terminator902/1
  CAN Unpack101/15 -> Bus Creator101/6  "Speed_Radial"
  CAN Unpack101/9 -> Terminator900/1
  CAN Unpack101/6 -> Terminator897/1
  CAN Unpack101/16 -> Bus Creator101/7  "CAN ID"
  CAN Unpack101/17 -> Bus Creator101/8  "Timestamp"
  Bus Creator101/1 -> Bus Creator1/101  "Data_100"
  CAN Unpack101/1 -> Bus Creator101/1  "AZ_Winkel"
  CAN Unpack102/3 -> Terminator903/1
  CAN Unpack102/2 -> Bus Creator102/2  "EL_Angle"
  CAN Unpack102/13 -> Terminator910/1
  CAN Unpack102/7 -> Terminator907/1
  CAN Unpack102/12 -> Bus Creator102/5  "Range"
  CAN Unpack102/10 -> Bus Creator102/3  "Mode_Signal"
  CAN Unpack102/4 -> Terminator904/1
  CAN Unpack102/5 -> Terminator905/1
  CAN Unpack102/8 -> Terminator908/1
  CAN Unpack102/11 -> Bus Creator102/4  "RCS"
  CAN Unpack102/14 -> Terminator911/1
  CAN Unpack102/15 -> Bus Creator102/6  "Speed_Radial"
  CAN Unpack102/9 -> Terminator909/1
  CAN Unpack102/6 -> Terminator906/1
  CAN Unpack102/16 -> Bus Creator102/7  "CAN ID"
  CAN Unpack102/17 -> Bus Creator102/8  "Timestamp"
  Bus Creator102/1 -> Bus Creator1/102  "Data_101"
  CAN Unpack102/1 -> Bus Creator102/1  "AZ_Winkel"
  CAN Unpack103/3 -> Terminator912/1
  CAN Unpack103/2 -> Bus Creator103/2  "EL_Angle"
  CAN Unpack103/13 -> Terminator919/1
  CAN Unpack103/7 -> Terminator916/1
  CAN Unpack103/12 -> Bus Creator103/5  "Range"
  CAN Unpack103/10 -> Bus Creator103/3  "Mode_Signal"
  CAN Unpack103/4 -> Terminator913/1
  CAN Unpack103/5 -> Terminator914/1
  CAN Unpack103/8 -> Terminator917/1
  CAN Unpack103/11 -> Bus Creator103/4  "RCS"
  CAN Unpack103/14 -> Terminator920/1
  CAN Unpack103/15 -> Bus Creator103/6  "Speed_Radial"
  CAN Unpack103/9 -> Terminator918/1
  CAN Unpack103/6 -> Terminator915/1
  CAN Unpack103/16 -> Bus Creator103/7  "CAN ID"
  CAN Unpack103/17 -> Bus Creator103/8  "Timestamp"
  Bus Creator103/1 -> Bus Creator1/103  "Data_102"
  CAN Unpack103/1 -> Bus Creator103/1  "AZ_Winkel"
  CAN Unpack104/3 -> Terminator921/1
  CAN Unpack104/2 -> Bus Creator104/2  "EL_Angle"
  CAN Unpack104/13 -> Terminator928/1
  CAN Unpack104/7 -> Terminator925/1
  CAN Unpack104/12 -> Bus Creator104/5  "Range"
  CAN Unpack104/10 -> Bus Creator104/3  "Mode_Signal"
  CAN Unpack104/4 -> Terminator922/1
  CAN Unpack104/5 -> Terminator923/1
  CAN Unpack104/8 -> Terminator926/1
  CAN Unpack104/11 -> Bus Creator104/4  "RCS"
  CAN Unpack104/14 -> Terminator929/1
  CAN Unpack104/15 -> Bus Creator104/6  "Speed_Radial"
  CAN Unpack104/9 -> Terminator927/1
  CAN Unpack104/6 -> Terminator924/1
  CAN Unpack104/16 -> Bus Creator104/7  "CAN ID"
  CAN Unpack104/17 -> Bus Creator104/8  "Timestamp"
  Bus Creator104/1 -> Bus Creator1/104  "Data_103"
  CAN Unpack104/1 -> Bus Creator104/1  "AZ_Winkel"
  CAN Unpack105/3 -> Terminator930/1
  CAN Unpack105/2 -> Bus Creator105/2  "EL_Angle"
  CAN Unpack105/13 -> Terminator937/1
  CAN Unpack105/7 -> Terminator934/1
  CAN Unpack105/12 -> Bus Creator105/5  "Range"
  CAN Unpack105/10 -> Bus Creator105/3  "Mode_Signal"
  CAN Unpack105/4 -> Terminator931/1
  CAN Unpack105/5 -> Terminator932/1
  CAN Unpack105/8 -> Terminator935/1
  CAN Unpack105/11 -> Bus Creator105/4  "RCS"
  CAN Unpack105/14 -> Terminator938/1
  CAN Unpack105/15 -> Bus Creator105/6  "Speed_Radial"
  CAN Unpack105/9 -> Terminator936/1
  CAN Unpack105/6 -> Terminator933/1
  CAN Unpack105/16 -> Bus Creator105/7  "CAN ID"
  CAN Unpack105/17 -> Bus Creator105/8  "Timestamp"
  Bus Creator105/1 -> Bus Creator1/105  "Data_104"
  CAN Unpack105/1 -> Bus Creator105/1  "AZ_Winkel"
  CAN Unpack106/3 -> Terminator939/1
  CAN Unpack106/2 -> Bus Creator106/2  "EL_Angle"
  CAN Unpack106/13 -> Terminator946/1
  CAN Unpack106/7 -> Terminator943/1
  CAN Unpack106/12 -> Bus Creator106/5  "Range"
  CAN Unpack106/10 -> Bus Creator106/3  "Mode_Signal"
  CAN Unpack106/4 -> Terminator940/1
  CAN Unpack106/5 -> Terminator941/1
  CAN Unpack106/8 -> Terminator944/1
  CAN Unpack106/11 -> Bus Creator106/4  "RCS"
  CAN Unpack106/14 -> Terminator947/1
  CAN Unpack106/15 -> Bus Creator106/6  "Speed_Radial"
  CAN Unpack106/9 -> Terminator945/1
  CAN Unpack106/6 -> Terminator942/1
  CAN Unpack106/16 -> Bus Creator106/7  "CAN ID"
  CAN Unpack106/17 -> Bus Creator106/8  "Timestamp"
  Bus Creator106/1 -> Bus Creator1/106  "Data_105"
  CAN Unpack106/1 -> Bus Creator106/1  "AZ_Winkel"
  CAN Unpack107/3 -> Terminator948/1
  CAN Unpack107/2 -> Bus Creator107/2  "EL_Angle"
  CAN Unpack107/13 -> Terminator955/1
  CAN Unpack107/7 -> Terminator952/1
  CAN Unpack107/12 -> Bus Creator107/5  "Range"
  CAN Unpack107/10 -> Bus Creator107/3  "Mode_Signal"
  CAN Unpack107/4 -> Terminator949/1
  CAN Unpack107/5 -> Terminator950/1
  CAN Unpack107/8 -> Terminator953/1
  CAN Unpack107/11 -> Bus Creator107/4  "RCS"
  CAN Unpack107/14 -> Terminator956/1
  CAN Unpack107/15 -> Bus Creator107/6  "Speed_Radial"
  CAN Unpack107/9 -> Terminator954/1
  CAN Unpack107/6 -> Terminator951/1
  CAN Unpack107/16 -> Bus Creator107/7  "CAN ID"
  CAN Unpack107/17 -> Bus Creator107/8  "Timestamp"
  Bus Creator107/1 -> Bus Creator1/107  "Data_106"
  CAN Unpack107/1 -> Bus Creator107/1  "AZ_Winkel"
  CAN Unpack108/3 -> Terminator957/1
  CAN Unpack108/2 -> Bus Creator108/2  "EL_Angle"
  CAN Unpack108/13 -> Terminator964/1
  CAN Unpack108/7 -> Terminator961/1
  CAN Unpack108/12 -> Bus Creator108/5  "Range"
  CAN Unpack108/10 -> Bus Creator108/3  "Mode_Signal"
  CAN Unpack108/4 -> Terminator958/1
  CAN Unpack108/5 -> Terminator959/1
  CAN Unpack108/8 -> Terminator962/1
  CAN Unpack108/11 -> Bus Creator108/4  "RCS"
  CAN Unpack108/14 -> Terminator965/1
  CAN Unpack108/15 -> Bus Creator108/6  "Speed_Radial"
  CAN Unpack108/9 -> Terminator963/1
  CAN Unpack108/6 -> Terminator960/1
  CAN Unpack108/16 -> Bus Creator108/7  "CAN ID"
  CAN Unpack108/17 -> Bus Creator108/8  "Timestamp"
  Bus Creator108/1 -> Bus Creator1/108  "Data_107"
  CAN Unpack108/1 -> Bus Creator108/1  "AZ_Winkel"
  CAN Unpack109/3 -> Terminator966/1
  CAN Unpack109/2 -> Bus Creator109/2  "EL_Angle"
  CAN Unpack109/13 -> Terminator973/1
  CAN Unpack109/7 -> Terminator970/1
  CAN Unpack109/12 -> Bus Creator109/5  "Range"
  CAN Unpack109/10 -> Bus Creator109/3  "Mode_Signal"
  CAN Unpack109/4 -> Terminator967/1
  CAN Unpack109/5 -> Terminator968/1
  CAN Unpack109/8 -> Terminator971/1
  CAN Unpack109/11 -> Bus Creator109/4  "RCS"
  CAN Unpack109/14 -> Terminator974/1
  CAN Unpack109/15 -> Bus Creator109/6  "Speed_Radial"
  CAN Unpack109/9 -> Terminator972/1
  CAN Unpack109/6 -> Terminator969/1
  CAN Unpack109/16 -> Bus Creator109/7  "CAN ID"
  CAN Unpack109/17 -> Bus Creator109/8  "Timestamp"
  Bus Creator109/1 -> Bus Creator1/109  "Data_108"
  CAN Unpack109/1 -> Bus Creator109/1  "AZ_Winkel"
  CAN Unpack110/3 -> Terminator975/1
  CAN Unpack110/2 -> Bus Creator110/2  "EL_Angle"
  CAN Unpack110/13 -> Terminator982/1
  CAN Unpack110/7 -> Terminator979/1
  CAN Unpack110/12 -> Bus Creator110/5  "Range"
  CAN Unpack110/10 -> Bus Creator110/3  "Mode_Signal"
  CAN Unpack110/4 -> Terminator976/1
  CAN Unpack110/5 -> Terminator977/1
  CAN Unpack110/8 -> Terminator980/1
  CAN Unpack110/11 -> Bus Creator110/4  "RCS"
  CAN Unpack110/14 -> Terminator983/1
  CAN Unpack110/15 -> Bus Creator110/6  "Speed_Radial"
  CAN Unpack110/9 -> Terminator981/1
  CAN Unpack110/6 -> Terminator978/1
  CAN Unpack110/16 -> Bus Creator110/7  "CAN ID"
  CAN Unpack110/17 -> Bus Creator110/8  "Timestamp"
  Bus Creator110/1 -> Bus Creator1/110  "Data_109"
  CAN Unpack110/1 -> Bus Creator110/1  "AZ_Winkel"
  CAN Unpack111/3 -> Terminator984/1
  CAN Unpack111/2 -> Bus Creator111/2  "EL_Angle"
  CAN Unpack111/13 -> Terminator991/1
  CAN Unpack111/7 -> Terminator988/1
  CAN Unpack111/12 -> Bus Creator111/5  "Range"
  CAN Unpack111/10 -> Bus Creator111/3  "Mode_Signal"
  CAN Unpack111/4 -> Terminator985/1
  CAN Unpack111/5 -> Terminator986/1
  CAN Unpack111/8 -> Terminator989/1
  CAN Unpack111/11 -> Bus Creator111/4  "RCS"
  CAN Unpack111/14 -> Terminator992/1
  CAN Unpack111/15 -> Bus Creator111/6  "Speed_Radial"
  CAN Unpack111/9 -> Terminator990/1
  CAN Unpack111/6 -> Terminator987/1
  CAN Unpack111/16 -> Bus Creator111/7  "CAN ID"
  CAN Unpack111/17 -> Bus Creator111/8  "Timestamp"
  Bus Creator111/1 -> Bus Creator1/111  "Data_110"
  CAN Unpack111/1 -> Bus Creator111/1  "AZ_Winkel"
  CAN Unpack112/3 -> Terminator993/1
  CAN Unpack112/2 -> Bus Creator112/2  "EL_Angle"
  CAN Unpack112/13 -> Terminator1000/1
  CAN Unpack112/7 -> Terminator997/1
  CAN Unpack112/12 -> Bus Creator112/5  "Range"
  CAN Unpack112/10 -> Bus Creator112/3  "Mode_Signal"
  CAN Unpack112/4 -> Terminator994/1
  CAN Unpack112/5 -> Terminator995/1
  CAN Unpack112/8 -> Terminator998/1
  CAN Unpack112/11 -> Bus Creator112/4  "RCS"
  CAN Unpack112/14 -> Terminator1001/1
  CAN Unpack112/15 -> Bus Creator112/6  "Speed_Radial"
  CAN Unpack112/9 -> Terminator999/1
  CAN Unpack112/6 -> Terminator996/1
  CAN Unpack112/16 -> Bus Creator112/7  "CAN ID"
  CAN Unpack112/17 -> Bus Creator112/8  "Timestamp"
  Bus Creator112/1 -> Bus Creator1/112  "Data_111"
  CAN Unpack112/1 -> Bus Creator112/1  "AZ_Winkel"
  CAN Unpack113/3 -> Terminator1002/1
  CAN Unpack113/2 -> Bus Creator113/2  "EL_Angle"
  CAN Unpack113/13 -> Terminator1009/1
  CAN Unpack113/7 -> Terminator1006/1
  CAN Unpack113/12 -> Bus Creator113/5  "Range"
  CAN Unpack113/10 -> Bus Creator113/3  "Mode_Signal"
  CAN Unpack113/4 -> Terminator1003/1
  CAN Unpack113/5 -> Terminator1004/1
  CAN Unpack113/8 -> Terminator1007/1
  CAN Unpack113/11 -> Bus Creator113/4  "RCS"
  CAN Unpack113/14 -> Terminator1010/1
  CAN Unpack113/15 -> Bus Creator113/6  "Speed_Radial"
  CAN Unpack113/9 -> Terminator1008/1
  CAN Unpack113/6 -> Terminator1005/1
  CAN Unpack113/16 -> Bus Creator113/7  "CAN ID"
  CAN Unpack113/17 -> Bus Creator113/8  "Timestamp"
  Bus Creator113/1 -> Bus Creator1/113  "Data_112"
  CAN Unpack113/1 -> Bus Creator113/1  "AZ_Winkel"
  CAN Unpack114/3 -> Terminator1011/1
  CAN Unpack114/2 -> Bus Creator114/2  "EL_Angle"
  CAN Unpack114/13 -> Terminator1018/1
  CAN Unpack114/7 -> Terminator1015/1
  CAN Unpack114/12 -> Bus Creator114/5  "Range"
  CAN Unpack114/10 -> Bus Creator114/3  "Mode_Signal"
  CAN Unpack114/4 -> Terminator1012/1
  CAN Unpack114/5 -> Terminator1013/1
  CAN Unpack114/8 -> Terminator1016/1
  CAN Unpack114/11 -> Bus Creator114/4  "RCS"
  CAN Unpack114/14 -> Terminator1019/1
  CAN Unpack114/15 -> Bus Creator114/6  "Speed_Radial"
  CAN Unpack114/9 -> Terminator1017/1
  CAN Unpack114/6 -> Terminator1014/1
  CAN Unpack114/16 -> Bus Creator114/7  "CAN ID"
  CAN Unpack114/17 -> Bus Creator114/8  "Timestamp"
  Bus Creator114/1 -> Bus Creator1/114  "Data_113"
  CAN Unpack114/1 -> Bus Creator114/1  "AZ_Winkel"
  CAN Unpack115/3 -> Terminator1020/1
  CAN Unpack115/2 -> Bus Creator115/2  "EL_Angle"
  CAN Unpack115/13 -> Terminator1027/1
  CAN Unpack115/7 -> Terminator1024/1
  CAN Unpack115/12 -> Bus Creator115/5  "Range"
  CAN Unpack115/10 -> Bus Creator115/3  "Mode_Signal"
  CAN Unpack115/4 -> Terminator1021/1
  CAN Unpack115/5 -> Terminator1022/1
  CAN Unpack115/8 -> Terminator1025/1
  CAN Unpack115/11 -> Bus Creator115/4  "RCS"
  CAN Unpack115/14 -> Terminator1028/1
  CAN Unpack115/15 -> Bus Creator115/6  "Speed_Radial"
  CAN Unpack115/9 -> Terminator1026/1
  CAN Unpack115/6 -> Terminator1023/1
  CAN Unpack115/16 -> Bus Creator115/7  "CAN ID"
  CAN Unpack115/17 -> Bus Creator115/8  "Timestamp"
  Bus Creator115/1 -> Bus Creator1/115  "Data_114"
  CAN Unpack115/1 -> Bus Creator115/1  "AZ_Winkel"
  CAN Unpack116/3 -> Terminator1029/1
  CAN Unpack116/2 -> Bus Creator116/2  "EL_Angle"
  CAN Unpack116/13 -> Terminator1036/1
  CAN Unpack116/7 -> Terminator1033/1
  CAN Unpack116/12 -> Bus Creator116/5  "Range"
  CAN Unpack116/10 -> Bus Creator116/3  "Mode_Signal"
  CAN Unpack116/4 -> Terminator1030/1
  CAN Unpack116/5 -> Terminator1031/1
  CAN Unpack116/8 -> Terminator1034/1
  CAN Unpack116/11 -> Bus Creator116/4  "RCS"
  CAN Unpack116/14 -> Terminator1037/1
  CAN Unpack116/15 -> Bus Creator116/6  "Speed_Radial"
  CAN Unpack116/9 -> Terminator1035/1
  CAN Unpack116/6 -> Terminator1032/1
  CAN Unpack116/16 -> Bus Creator116/7  "CAN ID"
  CAN Unpack116/17 -> Bus Creator116/8  "Timestamp"
  Bus Creator116/1 -> Bus Creator1/116  "Data_115"
  CAN Unpack116/1 -> Bus Creator116/1  "AZ_Winkel"
  CAN Unpack117/3 -> Terminator1038/1
  CAN Unpack117/2 -> Bus Creator117/2  "EL_Angle"
  CAN Unpack117/13 -> Terminator1045/1
  CAN Unpack117/7 -> Terminator1042/1
  CAN Unpack117/12 -> Bus Creator117/5  "Range"
  CAN Unpack117/10 -> Bus Creator117/3  "Mode_Signal"
  CAN Unpack117/4 -> Terminator1039/1
  CAN Unpack117/5 -> Terminator1040/1
  CAN Unpack117/8 -> Terminator1043/1
  CAN Unpack117/11 -> Bus Creator117/4  "RCS"
  CAN Unpack117/14 -> Terminator1046/1
  CAN Unpack117/15 -> Bus Creator117/6  "Speed_Radial"
  CAN Unpack117/9 -> Terminator1044/1
  CAN Unpack117/6 -> Terminator1041/1
  CAN Unpack117/16 -> Bus Creator117/7  "CAN ID"
  CAN Unpack117/17 -> Bus Creator117/8  "Timestamp"
  Bus Creator117/1 -> Bus Creator1/117  "Data_116"
  CAN Unpack117/1 -> Bus Creator117/1  "AZ_Winkel"
  CAN Unpack118/3 -> Terminator1047/1
  CAN Unpack118/2 -> Bus Creator118/2  "EL_Angle"
  CAN Unpack118/13 -> Terminator1054/1
  CAN Unpack118/7 -> Terminator1051/1
  CAN Unpack118/12 -> Bus Creator118/5  "Range"
  CAN Unpack118/10 -> Bus Creator118/3  "Mode_Signal"
  CAN Unpack118/4 -> Terminator1048/1
  CAN Unpack118/5 -> Terminator1049/1
  CAN Unpack118/8 -> Terminator1052/1
  CAN Unpack118/11 -> Bus Creator118/4  "RCS"
  CAN Unpack118/14 -> Terminator1055/1
  CAN Unpack118/15 -> Bus Creator118/6  "Speed_Radial"
  CAN Unpack118/9 -> Terminator1053/1
  CAN Unpack118/6 -> Terminator1050/1
  CAN Unpack118/16 -> Bus Creator118/7  "CAN ID"
  CAN Unpack118/17 -> Bus Creator118/8  "Timestamp"
  Bus Creator118/1 -> Bus Creator1/118  "Data_117"
  CAN Unpack118/1 -> Bus Creator118/1  "AZ_Winkel"
  CAN Unpack119/3 -> Terminator1056/1
  CAN Unpack119/2 -> Bus Creator119/2  "EL_Angle"
  CAN Unpack119/13 -> Terminator1063/1
  CAN Unpack119/7 -> Terminator1060/1
  CAN Unpack119/12 -> Bus Creator119/5  "Range"
  CAN Unpack119/10 -> Bus Creator119/3  "Mode_Signal"
  CAN Unpack119/4 -> Terminator1057/1
  CAN Unpack119/5 -> Terminator1058/1
  CAN Unpack119/8 -> Terminator1061/1
  CAN Unpack119/11 -> Bus Creator119/4  "RCS"
  CAN Unpack119/14 -> Terminator1064/1
  CAN Unpack119/15 -> Bus Creator119/6  "Speed_Radial"
  CAN Unpack119/9 -> Terminator1062/1
  CAN Unpack119/6 -> Terminator1059/1
  CAN Unpack119/16 -> Bus Creator119/7  "CAN ID"
  CAN Unpack119/17 -> Bus Creator119/8  "Timestamp"
  Bus Creator119/1 -> Bus Creator1/119  "Data_118"
  CAN Unpack119/1 -> Bus Creator119/1  "AZ_Winkel"
  CAN Unpack120/3 -> Terminator1065/1
  CAN Unpack120/2 -> Bus Creator120/2  "EL_Angle"
  CAN Unpack120/13 -> Terminator1072/1
  CAN Unpack120/7 -> Terminator1069/1
  CAN Unpack120/12 -> Bus Creator120/5  "Range"
  CAN Unpack120/10 -> Bus Creator120/3  "Mode_Signal"
  CAN Unpack120/4 -> Terminator1066/1
  CAN Unpack120/5 -> Terminator1067/1
  CAN Unpack120/8 -> Terminator1070/1
  CAN Unpack120/11 -> Bus Creator120/4  "RCS"
  CAN Unpack120/14 -> Terminator1073/1
  CAN Unpack120/15 -> Bus Creator120/6  "Speed_Radial"
  CAN Unpack120/9 -> Terminator1071/1
  CAN Unpack120/6 -> Terminator1068/1
  CAN Unpack120/16 -> Bus Creator120/7  "CAN ID"
  CAN Unpack120/17 -> Bus Creator120/8  "Timestamp"
  Bus Creator120/1 -> Bus Creator1/120  "Data_119"
  CAN Unpack120/1 -> Bus Creator120/1  "AZ_Winkel"
  CAN Unpack121/3 -> Terminator1074/1
  CAN Unpack121/2 -> Bus Creator121/2  "EL_Angle"
  CAN Unpack121/13 -> Terminator1081/1
  CAN Unpack121/7 -> Terminator1078/1
  CAN Unpack121/12 -> Bus Creator121/5  "Range"
  CAN Unpack121/10 -> Bus Creator121/3  "Mode_Signal"
  CAN Unpack121/4 -> Terminator1075/1
  CAN Unpack121/5 -> Terminator1076/1
  CAN Unpack121/8 -> Terminator1079/1
  CAN Unpack121/11 -> Bus Creator121/4  "RCS"
  CAN Unpack121/14 -> Terminator1082/1
  CAN Unpack121/15 -> Bus Creator121/6  "Speed_Radial"
  CAN Unpack121/9 -> Terminator1080/1
  CAN Unpack121/6 -> Terminator1077/1
  CAN Unpack121/16 -> Bus Creator121/7  "CAN ID"
  CAN Unpack121/17 -> Bus Creator121/8  "Timestamp"
  Bus Creator121/1 -> Bus Creator1/121  "Data_120"
  CAN Unpack121/1 -> Bus Creator121/1  "AZ_Winkel"
  CAN Unpack122/3 -> Terminator1083/1
  CAN Unpack122/2 -> Bus Creator122/2  "EL_Angle"
  CAN Unpack122/13 -> Terminator1090/1
  CAN Unpack122/7 -> Terminator1087/1
  CAN Unpack122/12 -> Bus Creator122/5  "Range"
  CAN Unpack122/10 -> Bus Creator122/3  "Mode_Signal"
  CAN Unpack122/4 -> Terminator1084/1
  CAN Unpack122/5 -> Terminator1085/1
  CAN Unpack122/8 -> Terminator1088/1
  CAN Unpack122/11 -> Bus Creator122/4  "RCS"
  CAN Unpack122/14 -> Terminator1091/1
  CAN Unpack122/15 -> Bus Creator122/6  "Speed_Radial"
  CAN Unpack122/9 -> Terminator1089/1
  CAN Unpack122/6 -> Terminator1086/1
  CAN Unpack122/16 -> Bus Creator122/7  "CAN ID"
  CAN Unpack122/17 -> Bus Creator122/8  "Timestamp"
  Bus Creator122/1 -> Bus Creator1/122  "Data_121"
  CAN Unpack122/1 -> Bus Creator122/1  "AZ_Winkel"
  CAN Unpack123/3 -> Terminator1092/1
  CAN Unpack123/2 -> Bus Creator123/2  "EL_Angle"
  CAN Unpack123/13 -> Terminator1099/1
  CAN Unpack123/7 -> Terminator1096/1
  CAN Unpack123/12 -> Bus Creator123/5  "Range"
  CAN Unpack123/10 -> Bus Creator123/3  "Mode_Signal"
  CAN Unpack123/4 -> Terminator1093/1
  CAN Unpack123/5 -> Terminator1094/1
  CAN Unpack123/8 -> Terminator1097/1
  CAN Unpack123/11 -> Bus Creator123/4  "RCS"
  CAN Unpack123/14 -> Terminator1100/1
  CAN Unpack123/15 -> Bus Creator123/6  "Speed_Radial"
  CAN Unpack123/9 -> Terminator1098/1
  CAN Unpack123/6 -> Terminator1095/1
  CAN Unpack123/16 -> Bus Creator123/7  "CAN ID"
  CAN Unpack123/17 -> Bus Creator123/8  "Timestamp"
  Bus Creator123/1 -> Bus Creator1/123  "Data_122"
  CAN Unpack123/1 -> Bus Creator123/1  "AZ_Winkel"
  CAN Unpack124/3 -> Terminator1101/1
  CAN Unpack124/2 -> Bus Creator124/2  "EL_Angle"
  CAN Unpack124/13 -> Terminator1108/1
  CAN Unpack124/7 -> Terminator1105/1
  CAN Unpack124/12 -> Bus Creator124/5  "Range"
  CAN Unpack124/10 -> Bus Creator124/3  "Mode_Signal"
  CAN Unpack124/4 -> Terminator1102/1
  CAN Unpack124/5 -> Terminator1103/1
  CAN Unpack124/8 -> Terminator1106/1
  CAN Unpack124/11 -> Bus Creator124/4  "RCS"
  CAN Unpack124/14 -> Terminator1109/1
  CAN Unpack124/15 -> Bus Creator124/6  "Speed_Radial"
  CAN Unpack124/9 -> Terminator1107/1
  CAN Unpack124/6 -> Terminator1104/1
  CAN Unpack124/16 -> Bus Creator124/7  "CAN ID"
  CAN Unpack124/17 -> Bus Creator124/8  "Timestamp"
  Bus Creator124/1 -> Bus Creator1/124  "Data_123"
  CAN Unpack124/1 -> Bus Creator124/1  "AZ_Winkel"
  CAN Unpack125/3 -> Terminator1110/1
  CAN Unpack125/2 -> Bus Creator125/2  "EL_Angle"
  CAN Unpack125/13 -> Terminator1117/1
  CAN Unpack125/7 -> Terminator1114/1
  CAN Unpack125/12 -> Bus Creator125/5  "Range"
  CAN Unpack125/10 -> Bus Creator125/3  "Mode_Signal"
  CAN Unpack125/4 -> Terminator1111/1
  CAN Unpack125/5 -> Terminator1112/1
  CAN Unpack125/8 -> Terminator1115/1
  CAN Unpack125/11 -> Bus Creator125/4  "RCS"
  CAN Unpack125/14 -> Terminator1118/1
  CAN Unpack125/15 -> Bus Creator125/6  "Speed_Radial"
  CAN Unpack125/9 -> Terminator1116/1
  CAN Unpack125/6 -> Terminator1113/1
  CAN Unpack125/16 -> Bus Creator125/7  "CAN ID"
  CAN Unpack125/17 -> Bus Creator125/8  "Timestamp"
  Bus Creator125/1 -> Bus Creator1/125  "Data_124"
  CAN Unpack125/1 -> Bus Creator125/1  "AZ_Winkel"
  CAN Unpack126/3 -> Terminator1119/1
  CAN Unpack126/2 -> Bus Creator126/2  "EL_Angle"
  CAN Unpack126/13 -> Terminator1126/1
  CAN Unpack126/7 -> Terminator1123/1
  CAN Unpack126/12 -> Bus Creator126/5  "Range"
  CAN Unpack126/10 -> Bus Creator126/3  "Mode_Signal"
  CAN Unpack126/4 -> Terminator1120/1
  CAN Unpack126/5 -> Terminator1121/1
  CAN Unpack126/8 -> Terminator1124/1
  CAN Unpack126/11 -> Bus Creator126/4  "RCS"
  CAN Unpack126/14 -> Terminator1127/1
  CAN Unpack126/15 -> Bus Creator126/6  "Speed_Radial"
  CAN Unpack126/9 -> Terminator1125/1
  CAN Unpack126/6 -> Terminator1122/1
  CAN Unpack126/16 -> Bus Creator126/7  "CAN ID"
  CAN Unpack126/17 -> Bus Creator126/8  "Timestamp"
  Bus Creator126/1 -> Bus Creator1/126  "Data_125"
  CAN Unpack126/1 -> Bus Creator126/1  "AZ_Winkel"
  CAN Unpack127/3 -> Terminator1128/1
  CAN Unpack127/2 -> Bus Creator127/2  "EL_Angle"
  CAN Unpack127/13 -> Terminator1135/1
  CAN Unpack127/7 -> Terminator1132/1
  CAN Unpack127/12 -> Bus Creator127/5  "Range"
  CAN Unpack127/10 -> Bus Creator127/3  "Mode_Signal"
  CAN Unpack127/4 -> Terminator1129/1
  CAN Unpack127/5 -> Terminator1130/1
  CAN Unpack127/8 -> Terminator1133/1
  CAN Unpack127/11 -> Bus Creator127/4  "RCS"
  CAN Unpack127/14 -> Terminator1136/1
  CAN Unpack127/15 -> Bus Creator127/6  "Speed_Radial"
  CAN Unpack127/9 -> Terminator1134/1
  CAN Unpack127/6 -> Terminator1131/1
  CAN Unpack127/16 -> Bus Creator127/7  "CAN ID"
  CAN Unpack127/17 -> Bus Creator127/8  "Timestamp"
  Bus Creator127/1 -> Bus Creator1/127  "Data_126"
  CAN Unpack127/1 -> Bus Creator127/1  "AZ_Winkel"
  CAN Unpack128/3 -> Terminator1137/1
  CAN Unpack128/2 -> Bus Creator128/2  "EL_Angle"
  CAN Unpack128/13 -> Terminator1144/1
  CAN Unpack128/7 -> Terminator1141/1
  CAN Unpack128/12 -> Bus Creator128/5  "Range"
  CAN Unpack128/10 -> Bus Creator128/3  "Mode_Signal"
  CAN Unpack128/4 -> Terminator1138/1
  CAN Unpack128/5 -> Terminator1139/1
  CAN Unpack128/8 -> Terminator1142/1
  CAN Unpack128/11 -> Bus Creator128/4  "RCS"
  CAN Unpack128/14 -> Terminator1145/1
  CAN Unpack128/15 -> Bus Creator128/6  "Speed_Radial"
  CAN Unpack128/9 -> Terminator1143/1
  CAN Unpack128/6 -> Terminator1140/1
  CAN Unpack128/16 -> Bus Creator128/7  "CAN ID"
  CAN Unpack128/17 -> Bus Creator128/8  "Timestamp"
  Bus Creator128/1 -> Bus Creator1/128  "Data_127"
  CAN Unpack128/1 -> Bus Creator128/1  "AZ_Winkel"
  CAN Unpack129/3 -> Terminator1146/1
  CAN Unpack129/2 -> Bus Creator129/2  "EL_Angle"
  CAN Unpack129/13 -> Terminator1153/1
  CAN Unpack129/7 -> Terminator1150/1
  CAN Unpack129/12 -> Bus Creator129/5  "Range"
  CAN Unpack129/10 -> Bus Creator129/3  "Mode_Signal"
  CAN Unpack129/4 -> Terminator1147/1
  CAN Unpack129/5 -> Terminator1148/1
  CAN Unpack129/8 -> Terminator1151/1
  CAN Unpack129/11 -> Bus Creator129/4  "RCS"
  CAN Unpack129/14 -> Terminator1154/1
  CAN Unpack129/15 -> Bus Creator129/6  "Speed_Radial"
  CAN Unpack129/9 -> Terminator1152/1
  CAN Unpack129/6 -> Terminator1149/1
  CAN Unpack129/16 -> Bus Creator129/7  "CAN ID"
  CAN Unpack129/17 -> Bus Creator129/8  "Timestamp"
  Bus Creator129/1 -> Bus Creator1/129  "Data_128"
  CAN Unpack129/1 -> Bus Creator129/1  "AZ_Winkel"
